simulink model "B_STUB"  (Simulink 8.1)
settings: Solver=ode1  StartTime=0.0  StopTime=1  FixedStep=Ts  MaxStep=1e-3  RelTol=1e-3
model workspace (MAT data in the model file):
  op_snapshot1 : opcond.OperatingPoint (value not decoded)
PostLoadFcn:
  | BANSHEE_init;
InitFcn:
  | BANSHEE_init;
values from neighbouring files (symbols this model uses):
  F2 = xlsread('F2_relay_banshee.xlsx')    [relay_settings_init.m]
  Ts = 100E-6    (= 0.0001)    [BANSHEE_init.m]
undefined symbols (not defined in the file or in its folder): cable_spec, Left, type, V
libraries: breaker_lib x20, relay_modbus_lib x19, rtio_generic_modbus x19, rtlab x18, cables_lib x11, transformer_lib x11, Load_lib x8, powerlib x6, ssn_lib x6, powerlib_extras x4, artemis x2, PQFV_lib x2
(part 1 of 2)
settings Model: ARTEMISmethode_block_infos=$$__separator__$$B_STUB/ARTEMIS Guide$$__separator__$$  Creator=RE25624  LastModifiedBy=re25624  BufferReuse=off
settings SolverCC: ZeroCrossAlgorithm=Adaptive
settings DataIOCC: ExternalInput=getinputstruct(op_snapshot1)  InitialState=getstatestruct(op_snapshot1)  LimitDataPoints=off  MaxDataPoints=90060  SignalLoggingSaveFormat=Dataset  SaveOutput=off  SignalLogging=off  DSMLogging=off  SaveTime=off  OutputSaveName=result
settings OptimizationCC: BlockReduction=off  OptimizeBlockIOStorage=off  BufferReuse=off  ExpressionFolding=off  LocalBlockOutputs=off
settings DebuggingCC: MaxConsecutiveZCsMsg=warning  IgnoredZcDiagnostic=none  SolverPrmCheckMsg=none  MultiTaskRateTransMsg=warning  FcnCallInpInsideContextMsg=EnableAllAsWarning  FrameProcessingCompatibilityMsg=error  ModelReferenceExtraNoncontSigs=warning  StrictBusMsg=None
settings ModelReferenceCC: UpdateModelReferenceTargets=IfOutOfDate
settings SFSimCC: SFSimEcho=off
settings GRTTargetCC: CodeReplacementLibrary=C89/C90 (ANSI)

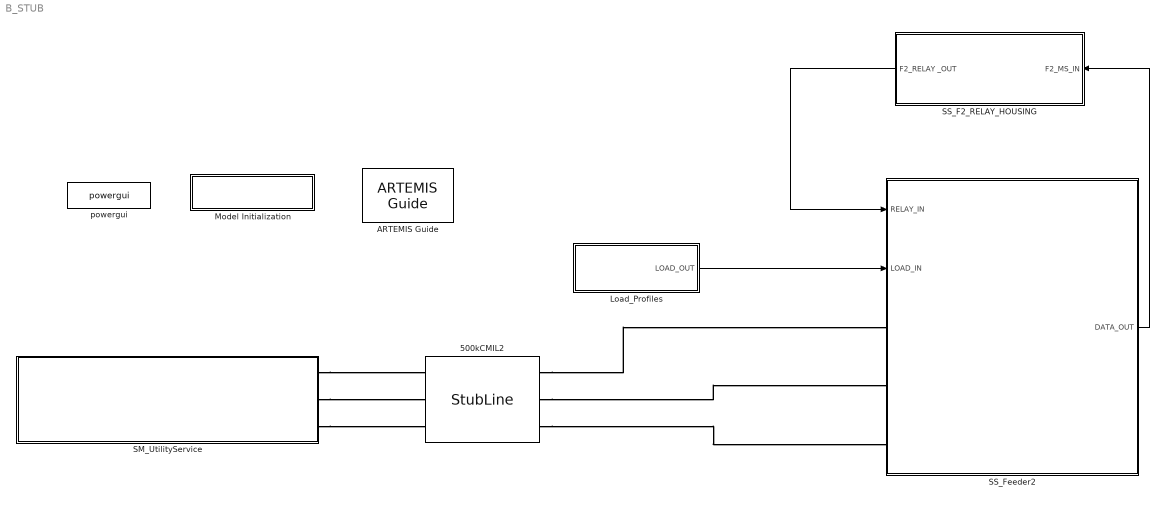
== system B_STUB ==
  500kCMIL2 : artemis/ARTEMIS/StubLine  Phases=3  pu=off  L=10000 * 9.43453e-08 / 1  Lpu=0.15  R=10000 * 2.28409e-5 / 1  Rpu=0.005  S_base=50e6/3  V_base=13.8e3/sqrt(3)  F_base=60  Ts=Ts
  ARTEMIS Guide : artemis/ARTEMIS/ARTEMIS Guide  Tag=FTSSmethode_opal_4hx0r99  Description=5.0_z1  lock=on  Ts=Ts  opt=art5  dyna=off  nb_perm=4  RT_fullcomp=off  ssn=on  ssn_itvc=off  ssn_ivic=off  ssn_ext=off  ssn_solver=Art5 with Backward Euler nodal interface  ssn_impulse=off  ssn_quasimpulse=off  ssn_impulse_loop=5  paraExtinctionThy=off  Thy_Impulse=on  dtc=Off  dtc_opt=normal  ao=on  simtype=off  ct_mac=off  lin_mov=off  lsp=[0.001 2]  spike_skip=Disabled  dtc_extra=1  dtc_sws=normal  dtc_pied=0.5  SPSRulesBlock=SPSRules  tre=on  ctmm=off  LF=off  dpl_type=ARTEMiS DPL  rlc_type=off  custom_type=off  para=on  ssn_ImpulseLoopBlockedStateUpdate=5  ssn_mov_iter_number=5  ssn_switch_iter_number=5
  Load_Profiles : Subsystem
  Model Initialization : Subsystem  AncestorBlock=artemis/Tools /Misc/Model Initialization  mask(Model Functions){InitFcnX=BANSHEE_init;, prel=off, posl=on, inif=on, strf=off}
      mask prompts: InitFcnX "Initialisation"; prel "Preload Function"; posl "PostLoad Function"; inif "InitFcn"; strf "StartFcn"
      mask init:
      | currentBlock = gcb;
      | root = bdroot(currentBlock);
      | 
      | if ~strcmp(get_param(root,'BlockDiagramType'),'library')
      |     if prel==1
      |         set_param(root, 'PreLoadFcn', InitFcnX);
      |     else
      |         set_param(root, 'PreLoadFcn', '');
      |     end
      |     if inif==1
      |         set_param(root, 'InitFcn', InitFcnX);
      |     else
      |         set_param(root, 'InitFcn', '');
      |     end
      |     if strf==1
      |         set_param(root, 'StartFcn', InitFcnX);
      |     else
      |         set_param(root, 'StartFcn', '');
      |     end
      |     if posl==1
      |         set_param(root, 'PostLoadFcn', InitFcnX);
      |     else
      |         set_param(root, 'PostLoadFcn', '');
      |     end
      | end
      | 
      | pos = get_param(currentBlock, 'Position');
      | width = pos(3) - pos(1); height = pos(4) - pos(2);
      | txt = [ upper(root) '\n' '- InitFcn. . . . . '  get_param(root, 'InitFcn') ];
      settings: CopyFcn=set_param(gcb,'LinkStatus','inactive')
      mask Display: text(5, height*0.5, txt, 'horizontalAlignment', 'left', 'verticalAlignment', 'middle') ;
  SM_UtilityService : Subsystem
  SS_F2_RELAY_HOUSING : Subsystem
  SS_Feeder2 : Subsystem
  powergui : powerlib/powergui  Priority=2  SimulationMode=Discrete  SolverType=Tustin  SampleTime=Ts  frequency=60  SPID=off  DisableSnubberDevices=off  DisableRonSwitches=off  DisableVfSwitches=off  SwTol=0  Interpol=off  DisplayEquations=off  frequencyindice=0  Pbase=100e6  ErrMax=1e-4  Iterations=50  UnitsV=kV  UnitsW=MW  FunctionMessages=off  echomessages=off  HookPort=off  EnableUseOfTLC=off  x0status=blocks  RestoreLinks=warning  ResistiveCurrentMeasurement=off  Frange=logspace(0,3,50)  Ylog=off  Xlog=off  ShowGrid=off  save=off  variable=ZData  structure=0  ZoomFFT=on  StartTime=0.0  cycles=2  DisplayStyle=off  fundamental=60  FreqAxis=off  MaxFrequency=1000  frequencyindicesteady=1  RmsSteady=1  display=off  Ts=0  methode=off
  wires:
  SS_F2_RELAY_HOUSING/1(F2_RELAY _OUT) -> SS_Feeder2/1(RELAY_IN)
  Load_Profiles/1(LOAD_OUT) -> SS_Feeder2/2(LOAD_IN)
  SS_Feeder2/1(DATA_OUT) -> SS_F2_RELAY_HOUSING/1(F2_MS_IN)
  connections:
  SM_UtilityService/RConn1 -- 500kCMIL2/LConn1
  SM_UtilityService/RConn2 -- 500kCMIL2/LConn2
  SM_UtilityService/RConn3 -- 500kCMIL2/LConn3
  500kCMIL2/RConn1 -- SS_Feeder2/LConn1
  500kCMIL2/RConn2 -- SS_Feeder2/LConn2
  500kCMIL2/RConn3 -- SS_Feeder2/LConn3

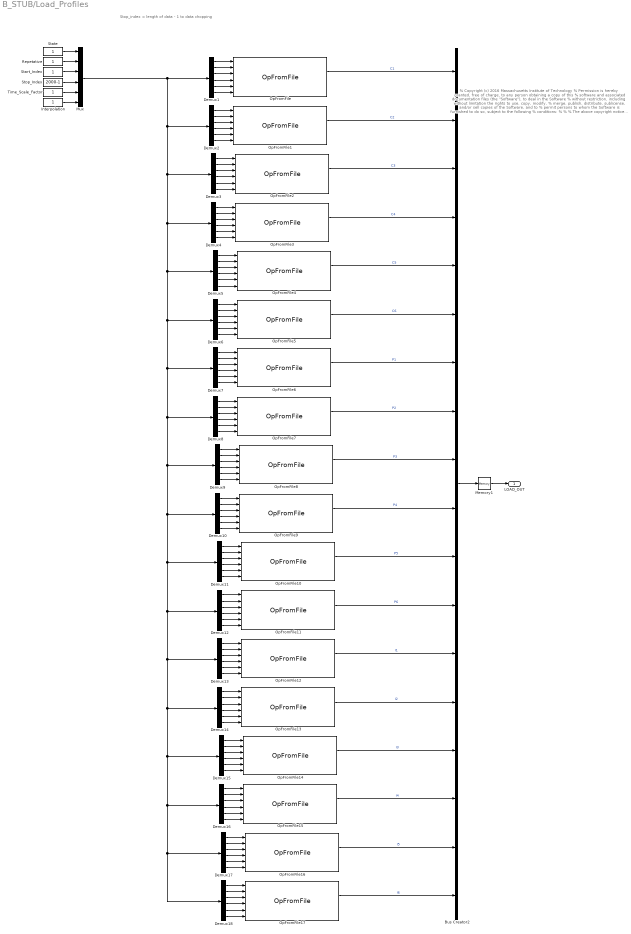
== system B_STUB/Load_Profiles ==
  note: Stop_index = length of data - 1 to data chopping
  note: % Copyright (c) 2016 Massachusetts Institute of Technology
      | % Permission is hereby granted, free of charge, to any person obtaining a copy of this
      | % software and associated documentation files (the "Software"), to deal in the Software
      | % without restriction, including without limitation the rights to use, copy, modify,
      | % merge, publish, distribute, sublicense, and/or sell copies of the Software, and to
      | % permit persons to whom the Software is furnished to do so, subject to the following
      | % conditions:
      | %
      | %
      | % The above copyright notice and this permission notice shall be included in
      | % all copies or substantial portions of the Software.
      | %
      | % THE SOFTWARE IS PROVIDED "AS IS", WITHOUT WARRANTY OF ANY KIND, EXPRESS OR IMPLIED,
      | % INCLUDING BUT NOT LIMITED TO THE WARRANTIES OF MERCHANTABILITY, FITNESS FOR A
      | % PARTICULAR PURPOSE AND NONINFRINGEMENT. IN NO EVENT SHALL THE AUTHORS OR COPYRIGHT
      | % HOLDERS BE LIABLE FOR ANY CLAIM, DAMAGES OR OTHER LIABILITY, WHETHER IN AN ACTION
      | % OF CONTRACT, TORT OR OTHERWISE, ARISING FROM, OUT OF OR IN CONNECTION WITH THE
      | % SOFTWARE OR THE USE OR OTHER DEALINGS IN THE SOFTWARE.
      | %
      | %
      | %%
  Bus Creator2 : BusCreator  Inputs=18
  Demux{1..18} (18 alike) : Demux  Outputs=6
  "Interpolation " : Constant
  Memory1 : Memory
  Mux : Mux  Inputs=6
  OpFromFile : rtlab/DataLogging/OpFromFile  filename_mode=Static (same filename all the time)  reload_mode=Next time model is paused (Real-Time)  init_file_id=0  filename=C1.mat  rtpath='./'  nrtpath='.\'  sample_time=0
  OpFromFile1 : rtlab/DataLogging/OpFromFile  filename_mode=Static (same filename all the time)  reload_mode=Next time model is paused (Real-Time)  init_file_id=0  filename=C2.mat  rtpath='./'  nrtpath='.\'  sample_time=0
  OpFromFile10 : rtlab/DataLogging/OpFromFile  filename_mode=Static (same filename all the time)  reload_mode=Next time model is paused (Real-Time)  init_file_id=0  filename=P5.mat  rtpath='./'  nrtpath='.\'  sample_time=0
  OpFromFile11 : rtlab/DataLogging/OpFromFile  filename_mode=Static (same filename all the time)  reload_mode=Next time model is paused (Real-Time)  init_file_id=0  filename=P6.mat  rtpath='./'  nrtpath='.\'  sample_time=0
  OpFromFile12 : rtlab/DataLogging/OpFromFile  filename_mode=Static (same filename all the time)  reload_mode=Next time model is paused (Real-Time)  init_file_id=0  filename=I1.mat  rtpath='./'  nrtpath='.\'  sample_time=0
  OpFromFile13 : rtlab/DataLogging/OpFromFile  filename_mode=Static (same filename all the time)  reload_mode=Next time model is paused (Real-Time)  init_file_id=0  filename=I2.mat  rtpath='./'  nrtpath='.\'  sample_time=0
  OpFromFile14 : rtlab/DataLogging/OpFromFile  filename_mode=Static (same filename all the time)  reload_mode=Next time model is paused (Real-Time)  init_file_id=0  filename=I3.mat  rtpath='./'  nrtpath='.\'  sample_time=0
  OpFromFile15 : rtlab/DataLogging/OpFromFile  filename_mode=Static (same filename all the time)  reload_mode=Next time model is paused (Real-Time)  init_file_id=0  filename=I4.mat  rtpath='./'  nrtpath='.\'  sample_time=0
  OpFromFile16 : rtlab/DataLogging/OpFromFile  filename_mode=Static (same filename all the time)  reload_mode=Next time model is paused (Real-Time)  init_file_id=0  filename=I5.mat  rtpath='./'  nrtpath='.\'  sample_time=0
  OpFromFile17 : rtlab/DataLogging/OpFromFile  filename_mode=Static (same filename all the time)  reload_mode=Next time model is paused (Real-Time)  init_file_id=0  filename=I6.mat  rtpath='./'  nrtpath='.\'  sample_time=0
  OpFromFile2 : rtlab/DataLogging/OpFromFile  filename_mode=Static (same filename all the time)  reload_mode=Next time model is paused (Real-Time)  init_file_id=0  filename=C3.mat  rtpath='./'  nrtpath='.\'  sample_time=0
  OpFromFile3 : rtlab/DataLogging/OpFromFile  filename_mode=Static (same filename all the time)  reload_mode=Next time model is paused (Real-Time)  init_file_id=0  filename=C4.mat  rtpath='./'  nrtpath='.\'  sample_time=0
  OpFromFile4 : rtlab/DataLogging/OpFromFile  filename_mode=Static (same filename all the time)  reload_mode=Next time model is paused (Real-Time)  init_file_id=0  filename=C5.mat  rtpath='./'  nrtpath='.\'  sample_time=0
  OpFromFile5 : rtlab/DataLogging/OpFromFile  filename_mode=Static (same filename all the time)  reload_mode=Next time model is paused (Real-Time)  init_file_id=0  filename=C6.mat  rtpath='./'  nrtpath='.\'  sample_time=0
  OpFromFile6 : rtlab/DataLogging/OpFromFile  filename_mode=Static (same filename all the time)  reload_mode=Next time model is paused (Real-Time)  init_file_id=0  filename=P1.mat  rtpath='./'  nrtpath='.\'  sample_time=0
  OpFromFile7 : rtlab/DataLogging/OpFromFile  filename_mode=Static (same filename all the time)  reload_mode=Next time model is paused (Real-Time)  init_file_id=0  filename=P2.mat  rtpath='./'  nrtpath='.\'  sample_time=0
  OpFromFile8 : rtlab/DataLogging/OpFromFile  filename_mode=Static (same filename all the time)  reload_mode=Next time model is paused (Real-Time)  init_file_id=0  filename=P3.mat  rtpath='./'  nrtpath='.\'  sample_time=0
  OpFromFile9 : rtlab/DataLogging/OpFromFile  filename_mode=Static (same filename all the time)  reload_mode=Next time model is paused (Real-Time)  init_file_id=0  filename=P4.mat  rtpath='./'  nrtpath='.\'  sample_time=0
  "Repetative " : Constant
  "Start_Index " : Constant
  "State " : Constant
  "Stop_Index " : Constant  Value=2000-1
  "Time_Scale_Factor " : Constant
  LOAD_OUT : Outport
  wires:
  Demux10/3 -> OpFromFile9/3
  Demux10/1 -> OpFromFile9/1
  Demux9/2 -> OpFromFile8/2
  Demux11/1 -> OpFromFile10/1
  Demux9/3 -> OpFromFile8/3
  Demux14/4 -> OpFromFile13/4
  Demux5/4 -> OpFromFile4/4
  Demux9/6 -> OpFromFile8/6
  Demux5/5 -> OpFromFile4/5
  Demux5/3 -> OpFromFile4/3
  Demux11/2 -> OpFromFile10/2
  Demux11/3 -> OpFromFile10/3
  Demux9/1 -> OpFromFile8/1
  Demux14/6 -> OpFromFile13/6
  Demux15/1 -> OpFromFile14/1
  Demux8/6 -> OpFromFile7/6
  Demux10/6 -> OpFromFile9/6
  Demux8/5 -> OpFromFile7/5
  OpFromFile3/2 -> Bus Creator2/4  "C4"
  Demux14/5 -> OpFromFile13/5
  OpFromFile5/2 -> Bus Creator2/6  "C6"
  OpFromFile4/2 -> Bus Creator2/5  "C5"
  "Interpolation "/1 -> Mux/6
  "Stop_Index "/1 -> Mux/4
  "Time_Scale_Factor "/1 -> Mux/5
  OpFromFile2/2 -> Bus Creator2/3  "C3"
  OpFromFile1/2 -> Bus Creator2/2  "C2"
  "Start_Index "/1 -> Mux/3
  OpFromFile/2 -> Bus Creator2/1  "C1"
  "State "/1 -> Mux/1
  "Repetative "/1 -> Mux/2
  Demux3/6 -> OpFromFile2/6
  Demux4/2 -> OpFromFile3/2
  Demux4/1 -> OpFromFile3/1
  Demux9/4 -> OpFromFile8/4
  Demux3/4 -> OpFromFile2/4
  Demux3/3 -> OpFromFile2/3
  Demux3/2 -> OpFromFile2/2
  Demux10/2 -> OpFromFile9/2
  Demux3/5 -> OpFromFile2/5
  Demux1/6 -> OpFromFile/6
  Demux1/5 -> OpFromFile/5
  Demux2/1 -> OpFromFile1/1
  Demux2/2 -> OpFromFile1/2
  Demux10/5 -> OpFromFile9/5
  Demux2/5 -> OpFromFile1/5
  Demux1/4 -> OpFromFile/4
  Demux2/3 -> OpFromFile1/3
  Demux2/4 -> OpFromFile1/4
  Demux3/1 -> OpFromFile2/1
  Demux10/4 -> OpFromFile9/4
  Demux2/6 -> OpFromFile1/6
  Demux1/3 -> OpFromFile/3
  Demux9/5 -> OpFromFile8/5
  Demux4/3 -> OpFromFile3/3
  Demux5/2 -> OpFromFile4/2
  Demux4/5 -> OpFromFile3/5
  Demux4/4 -> OpFromFile3/4
  Demux5/6 -> OpFromFile4/6
  Demux6/1 -> OpFromFile5/1
  Demux6/2 -> OpFromFile5/2
  Demux6/3 -> OpFromFile5/3
  Demux6/4 -> OpFromFile5/4
  Demux8/2 -> OpFromFile7/2
  Demux8/3 -> OpFromFile7/3
  Demux8/4 -> OpFromFile7/4
  Demux7/2 -> OpFromFile6/2
  Demux7/3 -> OpFromFile6/3
  Demux7/4 -> OpFromFile6/4
  Demux6/5 -> OpFromFile5/5
  Demux6/6 -> OpFromFile5/6
  Demux7/1 -> OpFromFile6/1
  Demux8/1 -> OpFromFile7/1
  Demux7/6 -> OpFromFile6/6
  Demux7/5 -> OpFromFile6/5
  Demux1/2 -> OpFromFile/2
  Demux1/1 -> OpFromFile/1
  Demux5/1 -> OpFromFile4/1
  Bus Creator2/1 -> Memory1/1
  Demux4/6 -> OpFromFile3/6
  Demux11/4 -> OpFromFile10/4
  Demux11/6 -> OpFromFile10/6
  Demux12/1 -> OpFromFile11/1
  Demux13/6 -> OpFromFile12/6
  Demux14/3 -> OpFromFile13/3
  Demux14/1 -> OpFromFile13/1
  Demux12/6 -> OpFromFile11/6
  Demux13/1 -> OpFromFile12/1
  Demux13/3 -> OpFromFile12/3
  Demux13/4 -> OpFromFile12/4
  Demux12/3 -> OpFromFile11/3
  Demux12/4 -> OpFromFile11/4
  Demux14/2 -> OpFromFile13/2
  OpFromFile11/2 -> Bus Creator2/12  "P6"
  Demux16/5 -> OpFromFile15/5
  Demux11/5 -> OpFromFile10/5
  Demux12/5 -> OpFromFile11/5
  Demux12/2 -> OpFromFile11/2
  Demux16/2 -> OpFromFile15/2
  Demux16/3 -> OpFromFile15/3
  Demux16/4 -> OpFromFile15/4
  Demux16/1 -> OpFromFile15/1
  Demux13/5 -> OpFromFile12/5
  Mux/1 -> Demux1/1, Demux2/1, Demux3/1, Demux4/1, Demux7/1, Demux8/1, Demux9/1, Demux10/1, Demux11/1, Demux12/1, Demux13/1, Demux14/1, Demux15/1, Demux16/1, Demux17/1, Demux18/1, Demux6/1, Demux5/1
  Demux15/3 -> OpFromFile14/3
  Demux15/4 -> OpFromFile14/4
  OpFromFile8/2 -> Bus Creator2/9  "P3"
  OpFromFile16/2 -> Bus Creator2/17  "I5"
  OpFromFile7/2 -> Bus Creator2/8  "P2"
  OpFromFile6/2 -> Bus Creator2/7  "P1"
  Demux18/6 -> OpFromFile17/6
  Demux18/5 -> OpFromFile17/5
  Demux18/4 -> OpFromFile17/4
  OpFromFile9/2 -> Bus Creator2/10  "P4"
  OpFromFile10/2 -> Bus Creator2/11  "P5"
  Demux15/5 -> OpFromFile14/5
  Demux15/6 -> OpFromFile14/6
  Demux18/3 -> OpFromFile17/3
  Demux17/5 -> OpFromFile16/5
  Demux18/1 -> OpFromFile17/1
  Demux18/2 -> OpFromFile17/2
  Demux17/6 -> OpFromFile16/6
  Demux17/2 -> OpFromFile16/2
  Demux17/3 -> OpFromFile16/3
  Demux17/1 -> OpFromFile16/1
  Demux17/4 -> OpFromFile16/4
  OpFromFile12/2 -> Bus Creator2/13  "I1"
  Demux15/2 -> OpFromFile14/2
  Demux13/2 -> OpFromFile12/2
  OpFromFile17/2 -> Bus Creator2/18  "I6"
  Demux16/6 -> OpFromFile15/6
  OpFromFile13/2 -> Bus Creator2/14  "I2"
  OpFromFile15/2 -> Bus Creator2/16  "I4"
  OpFromFile14/2 -> Bus Creator2/15  "I3"
  Memory1/1 -> LOAD_OUT/1

== system B_STUB/Model Initialization ==

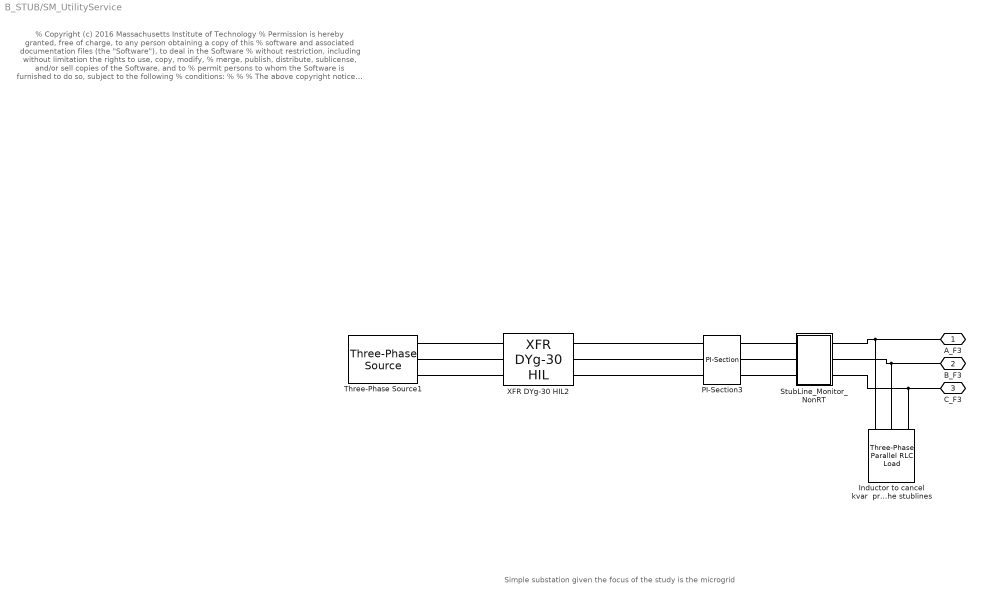
== system B_STUB/SM_UtilityService ==
  note: Simple substation given the focus of the study is the microgrid
  note: % Copyright (c) 2016 Massachusetts Institute of Technology
      | % Permission is hereby granted, free of charge, to any person obtaining a copy of this
      | % software and associated documentation files (the "Software"), to deal in the Software
      | % without restriction, including without limitation the rights to use, copy, modify,
      | % merge, publish, distribute, sublicense, and/or sell copies of the Software, and to
      | % permit persons to whom the Software is furnished to do so, subject to the following
      | % conditions:
      | %
      | %
      | % The above copyright notice and this permission notice shall be included in
      | % all copies or substantial portions of the Software.
      | %
      | % THE SOFTWARE IS PROVIDED "AS IS", WITHOUT WARRANTY OF ANY KIND, EXPRESS OR IMPLIED,
      | % INCLUDING BUT NOT LIMITED TO THE WARRANTIES OF MERCHANTABILITY, FITNESS FOR A
      | % PARTICULAR PURPOSE AND NONINFRINGEMENT. IN NO EVENT SHALL THE AUTHORS OR COPYRIGHT
      | % HOLDERS BE LIABLE FOR ANY CLAIM, DAMAGES OR OTHER LIABILITY, WHETHER IN AN ACTION
      | % OF CONTRACT, TORT OR OTHERWISE, ARISING FROM, OUT OF OR IN CONNECTION WITH THE
      | % SOFTWARE OR THE USE OR OTHER DEALINGS IN THE SOFTWARE.
      | %
      | %
      | %%
  Inductor to cancel kvar  produced by the stublines : powerlib/Elements/Three-Phase Parallel RLC Load  LConnTagsString=A|B|C  Configuration=Y (grounded)  NominalVoltage=13800  NominalFrequency=60  ActivePower=0  InductivePower=380e3  CapacitivePower=0  Measurements=None  LoadType=constant Z
  PI-Section3 : cables_lib/PI-Section  cable_spec=[cable_spec(13, :)]  line_length=500  parallel_sets=1
  StubLine_Monitor_NonRT : Subsystem  AncestorBlock=PQFV_lib/StubLine_Monitor_NonRT
  Three-Phase Source1 : powerlib/Electrical Sources/Three-Phase Source  Voltage=115000  PhaseAngle=0  Frequency=60  InternalConnection=Yg  SpecifyImpedance=on  Resistance=0.8929  Inductance=16.58e-3  ShortCircuitLevel=100e6  BaseVoltage=115000  XRratio=30  BusType=swing  Pref=0  Qref=0  Qmin=-inf  Qmax=inf
  XFR DYg-30 HIL2 : transformer_lib/XFR DYg-30 HIL  Rating=50000  Vp=115000  Vs=13800  Z=15  XR=30
  A_F3 : PMIOPort  Port=1  Side=Right
  B_F3 : PMIOPort  Port=2  Side=Right
  C_F3 : PMIOPort  Port=3  Side=Right
  connections:
  Three-Phase Source1/RConn3 -- XFR DYg-30 HIL2/LConn3
  Three-Phase Source1/RConn2 -- XFR DYg-30 HIL2/LConn2
  Three-Phase Source1/RConn1 -- XFR DYg-30 HIL2/LConn1
  StubLine_Monitor_NonRT/LConn1 -- PI-Section3/RConn1
  StubLine_Monitor_NonRT/LConn2 -- PI-Section3/RConn2
  StubLine_Monitor_NonRT/LConn3 -- PI-Section3/RConn3
  StubLine_Monitor_NonRT/RConn2 -- B_F3/RConn1 -- Inductor to cancel kvar  produced by the stublines/LConn2
  StubLine_Monitor_NonRT/RConn1 -- A_F3/RConn1 -- Inductor to cancel kvar  produced by the stublines/LConn1
  StubLine_Monitor_NonRT/RConn3 -- C_F3/RConn1 -- Inductor to cancel kvar  produced by the stublines/LConn3
  XFR DYg-30 HIL2/RConn3 -- PI-Section3/LConn3
  XFR DYg-30 HIL2/RConn2 -- PI-Section3/LConn2
  XFR DYg-30 HIL2/RConn1 -- PI-Section3/LConn1

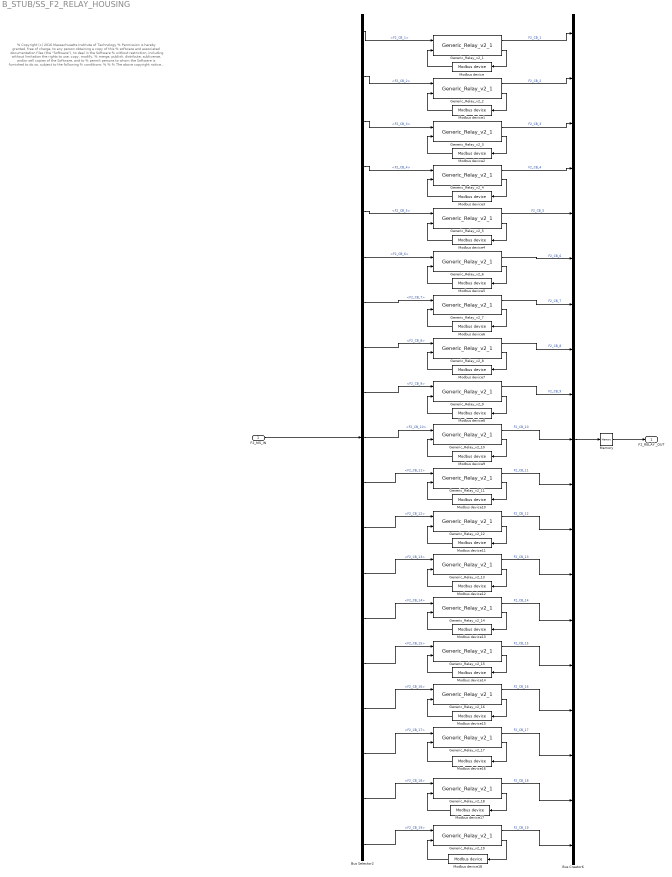
== system B_STUB/SS_F2_RELAY_HOUSING ==
  note: % Copyright (c) 2016 Massachusetts Institute of Technology
      | % Permission is hereby granted, free of charge, to any person obtaining a copy of this
      | % software and associated documentation files (the "Software"), to deal in the Software
      | % without restriction, including without limitation the rights to use, copy, modify,
      | % merge, publish, distribute, sublicense, and/or sell copies of the Software, and to
      | % permit persons to whom the Software is furnished to do so, subject to the following
      | % conditions:
      | %
      | %
      | % The above copyright notice and this permission notice shall be included in
      | % all copies or substantial portions of the Software.
      | %
      | % THE SOFTWARE IS PROVIDED "AS IS", WITHOUT WARRANTY OF ANY KIND, EXPRESS OR IMPLIED,
      | % INCLUDING BUT NOT LIMITED TO THE WARRANTIES OF MERCHANTABILITY, FITNESS FOR A
      | % PARTICULAR PURPOSE AND NONINFRINGEMENT. IN NO EVENT SHALL THE AUTHORS OR COPYRIGHT
      | % HOLDERS BE LIABLE FOR ANY CLAIM, DAMAGES OR OTHER LIABILITY, WHETHER IN AN ACTION
      | % OF CONTRACT, TORT OR OTHERWISE, ARISING FROM, OUT OF OR IN CONNECTION WITH THE
      | % SOFTWARE OR THE USE OR OTHER DEALINGS IN THE SOFTWARE.
      | %
      | %
      | %%
  F2_MS_IN : Inport
  Bus Creator6 : BusCreator  Inputs=19
  Bus Selector2 : BusSelector  OutputSignals=CB_DATA.F2_CB_1,CB_DATA.F2_CB_2,CB_DATA.F2_CB_3,CB_DATA.F2_CB_4,CB_DATA.F2_CB_5,CB_DATA.F2_CB_6,CB_DATA.F2_CB_7,CB_DATA.F2_CB_8,CB_DATA.F2_CB_9,CB_DATA.F2_CB_10,CB_DATA.F2_CB_11,CB_DATA.F2_CB_12,CB_DATA.F2_CB_13,CB_DATA.F2_CB_14,CB_DATA.F2_CB_15,CB_DATA.F2_CB_16,CB_DATA.F2_CB_17,CB_DATA.F2_CB_18,CB_DATA.F2_CB_19
  Generic_Relay_v2_1 : relay_modbus_lib/Generic_Relay_v2_1  Ts=Ts  relay_settings=[F2(1,:)]
  Generic_Relay_v2_10 : relay_modbus_lib/Generic_Relay_v2_1  Ts=Ts  relay_settings=[F2(10,:)]
  Generic_Relay_v2_11 : relay_modbus_lib/Generic_Relay_v2_1  Ts=Ts  relay_settings=[F2(11,:)]
  Generic_Relay_v2_12 : relay_modbus_lib/Generic_Relay_v2_1  Ts=Ts  relay_settings=[F2(12,:)]
  Generic_Relay_v2_13 : relay_modbus_lib/Generic_Relay_v2_1  Ts=Ts  relay_settings=[F2(13,:)]
  Generic_Relay_v2_14 : relay_modbus_lib/Generic_Relay_v2_1  Ts=Ts  relay_settings=[F2(14,:)]
  Generic_Relay_v2_15 : relay_modbus_lib/Generic_Relay_v2_1  Ts=Ts  relay_settings=[F2(15,:)]
  Generic_Relay_v2_16 : relay_modbus_lib/Generic_Relay_v2_1  Ts=Ts  relay_settings=[F2(16,:)]
  Generic_Relay_v2_17 : relay_modbus_lib/Generic_Relay_v2_1  Ts=Ts  relay_settings=[F2(17,:)]
  Generic_Relay_v2_18 : relay_modbus_lib/Generic_Relay_v2_1  Ts=Ts  relay_settings=[F2(18,:)]
  Generic_Relay_v2_19 : relay_modbus_lib/Generic_Relay_v2_1  Ts=Ts  relay_settings=[F2(19,:)]
  Generic_Relay_v2_2 : relay_modbus_lib/Generic_Relay_v2_1  Ts=Ts  relay_settings=[F2(2,:)]
  Generic_Relay_v2_3 : relay_modbus_lib/Generic_Relay_v2_1  Ts=Ts  relay_settings=[F2(3,:)]
  Generic_Relay_v2_4 : relay_modbus_lib/Generic_Relay_v2_1  Ts=Ts  relay_settings=[F2(4,:)]
  Generic_Relay_v2_5 : relay_modbus_lib/Generic_Relay_v2_1  Ts=Ts  relay_settings=[F2(5,:)]
  Generic_Relay_v2_6 : relay_modbus_lib/Generic_Relay_v2_1  Ts=Ts  relay_settings=[F2(6,:)]
  Generic_Relay_v2_7 : relay_modbus_lib/Generic_Relay_v2_1  Ts=Ts  relay_settings=[F2(7,:)]
  Generic_Relay_v2_8 : relay_modbus_lib/Generic_Relay_v2_1  Ts=Ts  relay_settings=[F2(8,:)]
  Generic_Relay_v2_9 : relay_modbus_lib/Generic_Relay_v2_1  Ts=Ts  relay_settings=[F2(9,:)]
  Memory : Memory
  Modbus device : rtio_generic_modbus/Modbus device  conf_name=F2_relay_cfg1.opal  conf_name_mask=F2_relay_cfg1.xls  sample_time=Ts
  Modbus device1 : rtio_generic_modbus/Modbus device  conf_name=F2_relay_cfg2.opal  conf_name_mask=F2_relay_cfg2.xls  sample_time=Ts
  Modbus device10 : rtio_generic_modbus/Modbus device  conf_name=F2_relay_cfg11.opal  conf_name_mask=F2_relay_cfg11.xls  sample_time=Ts
  Modbus device11 : rtio_generic_modbus/Modbus device  conf_name=F2_relay_cfg12.opal  conf_name_mask=F2_relay_cfg12.xls  sample_time=Ts
  Modbus device12 : rtio_generic_modbus/Modbus device  conf_name=F2_relay_cfg13.opal  conf_name_mask=F2_relay_cfg13.xls  sample_time=Ts
  Modbus device13 : rtio_generic_modbus/Modbus device  conf_name=F2_relay_cfg14.opal  conf_name_mask=F2_relay_cfg14.xls  sample_time=Ts
  Modbus device14 : rtio_generic_modbus/Modbus device  conf_name=F2_relay_cfg15.opal  conf_name_mask=F2_relay_cfg15.xls  sample_time=Ts
  Modbus device15 : rtio_generic_modbus/Modbus device  conf_name=F2_relay_cfg16.opal  conf_name_mask=F2_relay_cfg16.xls  sample_time=Ts
  Modbus device16 : rtio_generic_modbus/Modbus device  conf_name=F2_relay_cfg17.opal  conf_name_mask=F2_relay_cfg17.xls  sample_time=Ts
  Modbus device17 : rtio_generic_modbus/Modbus device  conf_name=F2_relay_cfg18.opal  conf_name_mask=F2_relay_cfg18.xls  sample_time=Ts
  Modbus device18 : rtio_generic_modbus/Modbus device  conf_name=F2_relay_cfg19.opal  conf_name_mask=F2_relay_cfg19.xls  sample_time=Ts
  Modbus device2 : rtio_generic_modbus/Modbus device  conf_name=F2_relay_cfg3.opal  conf_name_mask=F2_relay_cfg3.xls  sample_time=Ts
  Modbus device3 : rtio_generic_modbus/Modbus device  conf_name=F2_relay_cfg4.opal  conf_name_mask=F2_relay_cfg4.xls  sample_time=Ts
  Modbus device4 : rtio_generic_modbus/Modbus device  conf_name=F2_relay_cfg5.opal  conf_name_mask=F2_relay_cfg5.xls  sample_time=Ts
  Modbus device5 : rtio_generic_modbus/Modbus device  conf_name=F2_relay_cfg6.opal  conf_name_mask=F2_relay_cfg6.xls  sample_time=Ts
  Modbus device6 : rtio_generic_modbus/Modbus device  conf_name=F2_relay_cfg7.opal  conf_name_mask=F2_relay_cfg7.xls  sample_time=Ts
  Modbus device7 : rtio_generic_modbus/Modbus device  conf_name=F2_relay_cfg8.opal  conf_name_mask=F2_relay_cfg8.xls  sample_time=Ts
  Modbus device8 : rtio_generic_modbus/Modbus device  conf_name=F2_relay_cfg9.opal  conf_name_mask=F2_relay_cfg9.xls  sample_time=Ts
  Modbus device9 : rtio_generic_modbus/Modbus device  conf_name=F2_relay_cfg10.opal  conf_name_mask=F2_relay_cfg10.xls  sample_time=Ts
  F2_RELAY _OUT : Outport
  wires:
  Memory/1 -> F2_RELAY _OUT/1
  Bus Selector2/18 -> Generic_Relay_v2_18/1  "<F2_CB_18>"
  Bus Selector2/19 -> Generic_Relay_v2_19/1  "<F2_CB_19>"
  Generic_Relay_v2_19/1 -> Bus Creator6/19  "F2_CB_19"
  Generic_Relay_v2_18/1 -> Bus Creator6/18  "F2_CB_18"
  Generic_Relay_v2_18/2 -> Modbus device17/1
  Modbus device17/1 -> Generic_Relay_v2_18/2
  Generic_Relay_v2_19/2 -> Modbus device18/1
  Modbus device18/1 -> Generic_Relay_v2_19/2
  Bus Selector2/17 -> Generic_Relay_v2_17/1  "<F2_CB_17>"
  Generic_Relay_v2_17/1 -> Bus Creator6/17  "F2_CB_17"
  Generic_Relay_v2_6/1 -> Bus Creator6/6  "F2_CB_6"
  Generic_Relay_v2_5/1 -> Bus Creator6/5  "F2_CB_5"
  Generic_Relay_v2_4/1 -> Bus Creator6/4  "F2_CB_4"
  Generic_Relay_v2_3/1 -> Bus Creator6/3  "F2_CB_3"
  Generic_Relay_v2_2/1 -> Bus Creator6/2  "F2_CB_2"
  Generic_Relay_v2_7/1 -> Bus Creator6/7  "F2_CB_7"
  Generic_Relay_v2_8/1 -> Bus Creator6/8  "F2_CB_8"
  Generic_Relay_v2_9/1 -> Bus Creator6/9  "F2_CB_9"
  Generic_Relay_v2_10/1 -> Bus Creator6/10  "F2_CB_10"
  Generic_Relay_v2_11/1 -> Bus Creator6/11  "F2_CB_11"
  Generic_Relay_v2_16/1 -> Bus Creator6/16  "F2_CB_16"
  Generic_Relay_v2_15/1 -> Bus Creator6/15  "F2_CB_15"
  Generic_Relay_v2_14/1 -> Bus Creator6/14  "F2_CB_14"
  Generic_Relay_v2_13/1 -> Bus Creator6/13  "F2_CB_13"
  Generic_Relay_v2_12/1 -> Bus Creator6/12  "F2_CB_12"
  Bus Selector2/16 -> Generic_Relay_v2_16/1  "<F2_CB_16>"
  Bus Selector2/15 -> Generic_Relay_v2_15/1  "<F2_CB_15>"
  Bus Selector2/14 -> Generic_Relay_v2_14/1  "<F2_CB_14>"
  Bus Selector2/13 -> Generic_Relay_v2_13/1  "<F2_CB_13>"
  Bus Selector2/12 -> Generic_Relay_v2_12/1  "<F2_CB_12>"
  Bus Selector2/11 -> Generic_Relay_v2_11/1  "<F2_CB_11>"
  Bus Selector2/10 -> Generic_Relay_v2_10/1  "<F2_CB_10>"
  Bus Selector2/9 -> Generic_Relay_v2_9/1  "<F2_CB_9>"
  Bus Selector2/8 -> Generic_Relay_v2_8/1  "<F2_CB_8>"
  Bus Selector2/7 -> Generic_Relay_v2_7/1  "<F2_CB_7>"
  Bus Selector2/6 -> Generic_Relay_v2_6/1  "<F2_CB_6>"
  Bus Selector2/5 -> Generic_Relay_v2_5/1  "<F2_CB_5>"
  Bus Selector2/4 -> Generic_Relay_v2_4/1  "<F2_CB_4>"
  Bus Selector2/3 -> Generic_Relay_v2_3/1  "<F2_CB_3>"
  Bus Selector2/2 -> Generic_Relay_v2_2/1  "<F2_CB_2>"
  Generic_Relay_v2_1/1 -> Bus Creator6/1  "F2_CB_1"
  Bus Selector2/1 -> Generic_Relay_v2_1/1  "<F2_CB_1>"
  Bus Creator6/1 -> Memory/1
  Generic_Relay_v2_1/2 -> Modbus device/1
  Modbus device/1 -> Generic_Relay_v2_1/2
  Generic_Relay_v2_2/2 -> Modbus device1/1
  Modbus device1/1 -> Generic_Relay_v2_2/2
  Generic_Relay_v2_3/2 -> Modbus device2/1
  Modbus device2/1 -> Generic_Relay_v2_3/2
  Generic_Relay_v2_4/2 -> Modbus device3/1
  Modbus device3/1 -> Generic_Relay_v2_4/2
  Generic_Relay_v2_5/2 -> Modbus device4/1
  Modbus device4/1 -> Generic_Relay_v2_5/2
  Modbus device5/1 -> Generic_Relay_v2_6/2
  Generic_Relay_v2_6/2 -> Modbus device5/1
  Generic_Relay_v2_7/2 -> Modbus device6/1
  Modbus device6/1 -> Generic_Relay_v2_7/2
  Generic_Relay_v2_8/2 -> Modbus device7/1
  Modbus device7/1 -> Generic_Relay_v2_8/2
  Generic_Relay_v2_9/2 -> Modbus device8/1
  Modbus device8/1 -> Generic_Relay_v2_9/2
  Generic_Relay_v2_10/2 -> Modbus device9/1
  Modbus device9/1 -> Generic_Relay_v2_10/2
  Generic_Relay_v2_11/2 -> Modbus device10/1
  Modbus device10/1 -> Generic_Relay_v2_11/2
  Generic_Relay_v2_12/2 -> Modbus device11/1
  Modbus device11/1 -> Generic_Relay_v2_12/2
  Modbus device12/1 -> Generic_Relay_v2_13/2
  Generic_Relay_v2_13/2 -> Modbus device12/1
  Generic_Relay_v2_14/2 -> Modbus device13/1
  Modbus device13/1 -> Generic_Relay_v2_14/2
  Generic_Relay_v2_15/2 -> Modbus device14/1
  Modbus device14/1 -> Generic_Relay_v2_15/2
  Generic_Relay_v2_16/2 -> Modbus device15/1
  Modbus device15/1 -> Generic_Relay_v2_16/2
  Generic_Relay_v2_17/2 -> Modbus device16/1
  Modbus device16/1 -> Generic_Relay_v2_17/2
  F2_MS_IN/1 -> Bus Selector2/1

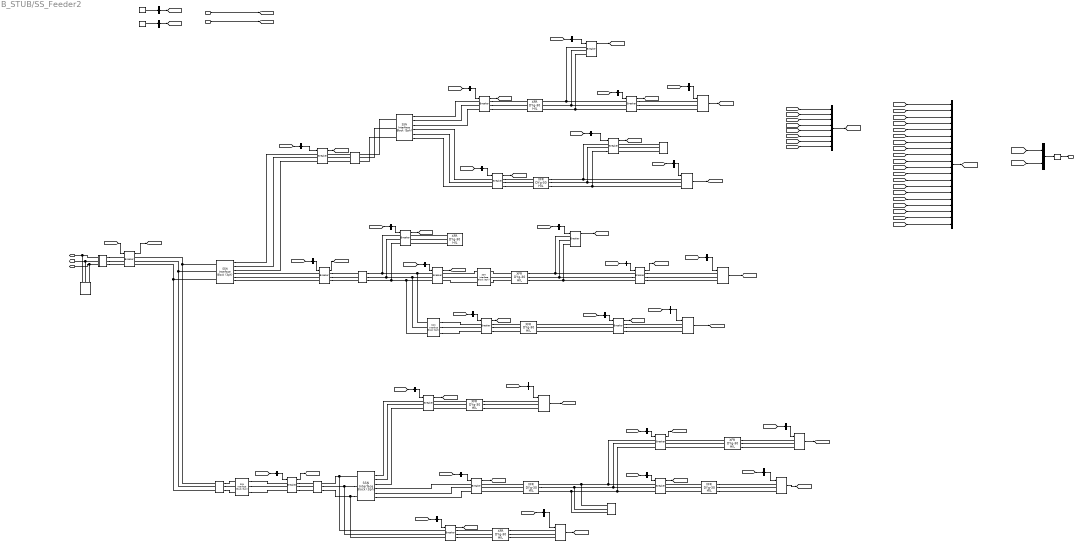
== system B_STUB/SS_Feeder2 ==
  note: Point-on-wave synchronisation voltage (3-phase) in PU - Using 13.8 kV
  note: % Copyright (c) 2016 Massachusetts Institute of Technology
      | % Permission is hereby granted, free of charge, to any person obtaining a copy of this
      | % software and associated documentation files (the "Software"), to deal in the Software
      | % without restriction, including without limitation the rights to use, copy, modify,
      | % merge, publish, distribute, sublicense, and/or sell copies of the Software, and to
      | % permit persons to whom the Software is furnished to do so, subject to the following
      | % conditions:
      | %
      | %
      | % The above copyright notice and this permission notice shall be included in
      | % all copies or substantial portions of the Software.
      | %
      | % THE SOFTWARE IS PROVIDED "AS IS", WITHOUT WARRANTY OF ANY KIND, EXPRESS OR IMPLIED,
      | % INCLUDING BUT NOT LIMITED TO THE WARRANTIES OF MERCHANTABILITY, FITNESS FOR A
      | % PARTICULAR PURPOSE AND NONINFRINGEMENT. IN NO EVENT SHALL THE AUTHORS OR COPYRIGHT
      | % HOLDERS BE LIABLE FOR ANY CLAIM, DAMAGES OR OTHER LIABILITY, WHETHER IN AN ACTION
      | % OF CONTRACT, TORT OR OTHERWISE, ARISING FROM, OUT OF OR IN CONNECTION WITH THE
      | % SOFTWARE OR THE USE OR OTHER DEALINGS IN THE SOFTWARE.
      | %
      | %
      | %%
  note: PV SYSTEM
  note: BATT SYSTEM
  note: connect to F3
  note: connect to F3
  note: connect to F3
  RELAY_IN : Inport
  LOAD_IN : Inport  Port=2
  1000 kVA1 : transformer_lib/XFR DYg-30 HIL  Rating=1000  Vp=13800  Vs=480  Z=5.56  XR=4.49
  1000 kVA2 : transformer_lib/XFR DYg-30 HIL  Rating=1000  Vp=13800  Vs=480  Z=5.56  XR=5.49
  1500 kVA : transformer_lib/XFR DYg-30 HIL  Rating=1500  Vp=13800  Vs=480  Z=5.56  XR=5.51
  2000 kVA2 : transformer_lib/XFR DYg-30 HIL  Rating=2000  Vp=13800  Vs=480  Z=5.75  XR=5.7
  2000 kVA3 : transformer_lib/XFR DYg-30 HIL  Rating=2000  Vp=13800  Vs=480  Z=5.75  XR=5.7
  2500 kVA : transformer_lib/XFR DYg-30 HIL  Rating=2500  Vp=13800  Vs=480  Z=5.56  XR=5.52
  2500 kVA1 : transformer_lib/XFR DYg-30 HIL  Rating=2500  Vp=13800  Vs=480  Z=5.56  XR=5.52
  3750 kVA : transformer_lib/XFR DYg-30 HIL  Rating=3750  Vp=13800  Vs=4160  Z=4.75  XR=11.4
  500 kVA : transformer_lib/XFR DYg-30 HIL  Rating=500  Vp=13800  Vs=208  Z=5  XR=4.9
  5000 kVA : transformer_lib/XFR DYg-30 HIL  Rating=5000  Vp=13800  Vs=480  Z=5.50  XR=5.44
  Bus Creator : BusCreator  Inputs=1
  Bus Creator1 : BusCreator  Inputs=1
  Bus Creator2 : BusCreator  Inputs=2
  Bus Creator3 : BusCreator  Inputs=8
  Bus Creator5 : BusCreator  Inputs=20
  Bus Selector1 : BusSelector  OutputSignals=F2_CB_4
  Bus Selector10 : BusSelector  OutputSignals=I4
  Bus Selector11 : BusSelector  OutputSignals=F2_CB_11
  Bus Selector12 : BusSelector  OutputSignals=F2_CB_15
  Bus Selector13 : BusSelector  OutputSignals=F2_CB_3
  Bus Selector14 : BusSelector  OutputSignals=F2_CB_14
  Bus Selector15 : BusSelector  OutputSignals=F2_CB_17
  Bus Selector16 : BusSelector  OutputSignals=F2_CB_16
  Bus Selector17 : BusSelector  OutputSignals=F2_CB_13
  Bus Selector18 : BusSelector  OutputSignals=F2_CB_10
  Bus Selector19 : BusSelector  OutputSignals=F2_CB_9
  Bus Selector2 : BusSelector  OutputSignals=F2_CB_2
  Bus Selector20 : BusSelector  OutputSignals=F2_CB_12
  Bus Selector21 : BusSelector  OutputSignals=F2_CB_5
  Bus Selector22 : BusSelector  OutputSignals=F2_CB_7
  Bus Selector23 : BusSelector  OutputSignals=F2_CB_8
  Bus Selector24 : BusSelector  OutputSignals=F2_CB_6
  Bus Selector25 : BusSelector  OutputSignals=F2_CB_1
  Bus Selector26 : BusSelector  OutputSignals=F2_CB_18
  Bus Selector27 : BusSelector  OutputSignals=F2_CB_19
  Bus Selector3 : BusSelector  OutputSignals=P5
  Bus Selector4 : BusSelector  OutputSignals=C4
  Bus Selector5 : BusSelector  OutputSignals=I5
  Bus Selector6 : BusSelector  OutputSignals=P2
  Bus Selector7 : BusSelector  OutputSignals=C3
  Bus Selector8 : BusSelector  OutputSignals=P3
  Bus Selector9 : BusSelector  OutputSignals=I3
  C1 : cables_lib/PI-Section  cable_spec=[cable_spec(11, :)]  line_length=10  parallel_sets=1
  C201 : cables_lib/PI-Section  cable_spec=[cable_spec(11, :)]  line_length=5500  parallel_sets=1
  C202 : cables_lib/PI-Section  cable_spec=[cable_spec(13, :)]  line_length=2000  parallel_sets=1
  C203 : cables_lib/PI-Section  cable_spec=[cable_spec(13, :)]  line_length=3000  parallel_sets=1
  C205 : cables_lib/PI-Section  cable_spec=[cable_spec(6, :)]  line_length=1500  parallel_sets=2
  C206 : cables_lib/PI-Section  cable_spec=[cable_spec(6, :)]  line_length=1500  parallel_sets=2
  CB closed : Constant
  CB open : Constant  Value=0
  Critical_3 : Load_lib/Dynamic_Load  V=460  Ts=Ts
  Critical_4 : Load_lib/Dynamic_Load  V=460  Ts=Ts
  F2_CB_{1..19} (19 alike) : breaker_lib/Breaker  Ts=Ts  mech_delay=cb_mech_delay
  F2_PCC : breaker_lib/Breaker  Ts=Ts  mech_delay=cb_mech_delay
  Interruptible_3 : Load_lib/Dynamic_Load  V=208  Ts=Ts
  Interruptible_4 : Load_lib/Dynamic_Load  V=460  Ts=Ts
  Interruptible_5 : Load_lib/Dynamic_Load  V=460  Ts=Ts
  Memory : Memory
  Priority_2 : Load_lib/Dynamic_Load  V=460  Ts=Ts
  Priority_3 : Load_lib/Dynamic_Load  V=460  Ts=Ts
  Priority_5 : Load_lib/Dynamic_Load  V=460  Ts=Ts
  SSN Interface Block (3ph)1 : ssn_lib/SSN Interface Block (3ph)  nb_phase=3  nb_port=3  p1_type=V-type(Left)  p2_type=V-type (Right)  p3_type=V-type (Right)  p4_type=V-type(Left)  p5_type=V-type(Left)  p6_type=V-type(Left)  p7_type=V-type(Left)  p8_type=V-type(Left)  p9_type=V-type(Left)  p10_type=V-type(Left)  p11_type=V-type(Left)  p12_type=V-type(Left)  p13_type=V-type(Left)  p14_type=V-type(Left)  p15_type=V-type(Left)  p16_type=V-type(Left)  I_port_shunt_resistance=1e9
  SSN Interface Block (3ph)10 : ssn_lib/SSN Interface Block (3ph)  nb_phase=3  nb_port=2  p1_type=V-type(Left)  p2_type=V-type (Right)  p3_type=V-type(Left)  p4_type=V-type(Left)  p5_type=V-type(Left)  p6_type=V-type(Left)  p7_type=V-type(Left)  p8_type=V-type(Left)  p9_type=V-type(Left)  p10_type=V-type(Left)  p11_type=V-type(Left)  p12_type=V-type(Left)  p13_type=V-type(Left)  p14_type=V-type(Left)  p15_type=V-type(Left)  p16_type=V-type(Left)  I_port_shunt_resistance=1e9
  SSN Interface Block (3ph)2 : ssn_lib/SSN Interface Block (3ph)  nb_phase=3  nb_port=3  p1_type=V-type(Left)  p2_type=V-type (Right)  p3_type=V-type (Right)  p4_type=V-type(Left)  p5_type=V-type(Left)  p6_type=V-type(Left)  p7_type=V-type(Left)  p8_type=V-type(Left)  p9_type=V-type(Left)  p10_type=V-type(Left)  p11_type=V-type(Left)  p12_type=V-type(Left)  p13_type=V-type(Left)  p14_type=V-type(Left)  p15_type=V-type(Left)  p16_type=V-type(Left)  I_port_shunt_resistance=1e9
  SSN Interface Block (3ph)3 : ssn_lib/SSN Interface Block (3ph)  nb_phase=3  nb_port=2  p1_type=V-type(Left)  p2_type=V-type (Right)  p3_type=V-type(Left)  p4_type=V-type(Left)  p5_type=V-type(Left)  p6_type=V-type(Left)  p7_type=V-type(Left)  p8_type=V-type(Left)  p9_type=V-type(Left)  p10_type=V-type(Left)  p11_type=V-type(Left)  p12_type=V-type(Left)  p13_type=V-type(Left)  p14_type=V-type(Left)  p15_type=V-type(Left)  p16_type=V-type(Left)  I_port_shunt_resistance=1e9
  SSN Interface Block (3ph)4 : ssn_lib/SSN Interface Block (3ph)  nb_phase=3  nb_port=3  p1_type=V-type(Left)  p2_type=V-type (Right)  p3_type=V-type (Right)  p4_type=V-type(Left)  p5_type=V-type(Left)  p6_type=V-type(Left)  p7_type=V-type(Left)  p8_type=V-type(Left)  p9_type=V-type(Left)  p10_type=V-type(Left)  p11_type=V-type(Left)  p12_type=V-type(Left)  p13_type=V-type(Left)  p14_type=V-type(Left)  p15_type=V-type(Left)  p16_type=V-type(Left)  I_port_shunt_resistance=1e9
  SSN Interface Block (3ph)9 : ssn_lib/SSN Interface Block (3ph)  nb_phase=3  nb_port=2  p1_type=V-type(Left)  p2_type=V-type (Right)  p3_type=V-type(Left)  p4_type=V-type(Left)  p5_type=V-type(Left)  p6_type=V-type(Left)  p7_type=V-type(Left)  p8_type=V-type(Left)  p9_type=V-type(Left)  p10_type=V-type(Left)  p11_type=V-type(Left)  p12_type=V-type(Left)  p13_type=V-type(Left)  p14_type=V-type(Left)  p15_type=V-type(Left)  p16_type=V-type(Left)  I_port_shunt_resistance=1e9
  StubLine_Monitor_NonRT : Subsystem  AncestorBlock=PQFV_lib/StubLine_Monitor_NonRT
  Three-Phase Parallel RLC Load : powerlib/Elements/Three-Phase Parallel RLC Load  LConnTagsString=A|B|C  Configuration=Y (grounded)  NominalVoltage=13800  NominalFrequency=60  ActivePower=0  InductivePower=380e3  CapacitivePower=0  Measurements=None  LoadType=constant Z
  A_PCC : PMIOPort  Port=1  Side=Left
  B_PCC : PMIOPort  Port=2  Side=Left
  C_PCC : PMIOPort  Port=3  Side=Left
  DATA_OUT : Outport
  wires:
  [LOAD_DATA] -> Bus Creator2/2  "LOAD_DATA"
  [CB_DATA] -> Bus Creator2/1  "CB_DATA"
  Bus Creator5/1 -> [CB_DATA]
  Bus Creator2/1 -> Memory/1
  Memory/1 -> DATA_OUT/1
  Bus Selector27/1 -> F2_CB_19/1  "<F2_CB_19>"
  [RELAY_IN] -> Bus Selector27/1
  F2_CB_19/1 -> [F2_CB_19]
  [F2_CB_19] -> Bus Creator5/19  "F2_CB_19"
  [F2_CB_18] -> Bus Creator5/18  "F2_CB_18"
  Bus Selector26/1 -> F2_CB_18/1  "<F2_CB_18>"
  [RELAY_IN] -> Bus Selector26/1
  F2_CB_18/1 -> [F2_CB_18]
  Bus Selector1/1 -> F2_CB_4/1  "<F2_CB_4>"
  [RELAY_IN] -> Bus Selector1/1
  F2_CB_4/1 -> [F2_CB_4]
  [F2_PCC] -> Bus Creator5/20  "F2_PCC"
  F2_PCC/1 -> [F2_PCC]
  F2_CB_16/1 -> [F2_CB_16]
  F2_CB_12/1 -> [F2_CB_12]
  Bus Selector15/1 -> F2_CB_17/1  "<F2_CB_17>"
  [F2_CB_17] -> Bus Creator5/17  "F2_CB_17"
  Bus Selector23/1 -> F2_CB_8/1  "<F2_CB_8>"
  Bus Selector24/1 -> F2_CB_6/1  "<F2_CB_6>"
  Bus Selector22/1 -> F2_CB_7/1  "<F2_CB_7>"
  Bus Selector21/1 -> F2_CB_5/1  "<F2_CB_5>"
  Bus Selector25/1 -> F2_CB_1/1  "<F2_CB_1>"
  Bus Selector12/1 -> F2_CB_15/1  "<F2_CB_15>"
  Bus Selector16/1 -> F2_CB_16/1  "<F2_CB_16>"
  Bus Selector14/1 -> F2_CB_14/1  "<F2_CB_14>"
  Bus Selector20/1 -> F2_CB_12/1  "<F2_CB_12>"
  Bus Selector17/1 -> F2_CB_13/1  "<F2_CB_13>"
  Bus Selector19/1 -> F2_CB_9/1  "<F2_CB_9>"
  Bus Selector18/1 -> F2_CB_10/1  "<F2_CB_10>"
  Bus Selector11/1 -> F2_CB_11/1  "<F2_CB_11>"
  Bus Selector2/1 -> F2_CB_2/1  "<F2_CB_2>"
  [RELAY_IN] -> Bus Selector25/1
  [RELAY_IN] -> Bus Selector24/1
  [RELAY_IN] -> Bus Selector23/1
  [RELAY_IN] -> Bus Selector22/1
  [RELAY_IN] -> Bus Selector21/1
  [RELAY_IN] -> Bus Selector20/1
  [RELAY_IN] -> Bus Selector19/1
  [RELAY_IN] -> Bus Selector18/1
  [RELAY_IN] -> Bus Selector17/1
  [RELAY_IN] -> Bus Selector16/1
  [RELAY_IN] -> Bus Selector15/1
  [RELAY_IN] -> Bus Selector14/1
  [RELAY_IN] -> Bus Selector12/1
  [RELAY_IN] -> Bus Selector11/1
  [RELAY_IN] -> Bus Selector2/1
  [RELAY_IN] -> Bus Selector13/1
  Bus Selector13/1 -> F2_CB_3/1  "<F2_CB_3>"
  RELAY_IN/1 -> [RELAY_IN]
  [F2_CB_16] -> Bus Creator5/16  "F2_CB_16"
  [F2_CB_15] -> Bus Creator5/15  "F2_CB_15"
  [F2_CB_13] -> Bus Creator5/13  "F2_CB_13"
  [F2_CB_10] -> Bus Creator5/10  "F2_CB_10"
  [F2_CB_12] -> Bus Creator5/12  "F2_CB_12"
  [F2_CB_8] -> Bus Creator5/8  "F2_CB_8"
  [F2_CB_5] -> Bus Creator5/5  "F2_CB_5"
  [F2_CB_14] -> Bus Creator5/14  "F2_CB_14"
  [F2_CB_11] -> Bus Creator5/11  "F2_CB_11"
  [F2_CB_7] -> Bus Creator5/7  "F2_CB_7"
  [F2_CB_9] -> Bus Creator5/9  "F2_CB_9"
  [F2_CB_4] -> Bus Creator5/4  "F2_CB_4"
  [F2_CB_6] -> Bus Creator5/6  "F2_CB_6"
  [F2_CB_3] -> Bus Creator5/3  "F2_CB_3"
  [F2_CB_2] -> Bus Creator5/2  "F2_CB_2"
  [F2_CB_1] -> Bus Creator5/1  "F2_CB_1"
  F2_CB_13/1 -> [F2_CB_13]
  F2_CB_10/1 -> [F2_CB_10]
  F2_CB_14/1 -> [F2_CB_14]
  F2_CB_17/1 -> [F2_CB_17]
  F2_CB_15/1 -> [F2_CB_15]
  F2_CB_11/1 -> [F2_CB_11]
  F2_CB_3/1 -> [F2_CB_3]
  F2_CB_9/1 -> [F2_CB_9]
  F2_CB_8/1 -> [F2_CB_8]
  F2_CB_5/1 -> [F2_CB_5]
  F2_CB_7/1 -> [F2_CB_7]
  F2_CB_6/1 -> [F2_CB_6]
  F2_CB_1/1 -> [F2_CB_1]
  F2_CB_2/1 -> [F2_CB_2]
  [LOAD_P5] -> Bus Creator3/8  "F2_P5"
  [LOAD_P3] -> Bus Creator3/7  "F2_P3"
  [LOAD_I3] -> Bus Creator3/3  "F2_I3"
  [LOAD_C4] -> Bus Creator3/2  "F2_C4"
  [LOAD_I5] -> Bus Creator3/5  "F2_I5"
  [LOAD_P2] -> Bus Creator3/6  "F2_P2"
  [LOAD_I4] -> Bus Creator3/4  "F2_I4"
  Bus Creator3/1 -> [LOAD_DATA]  "LOAD"
  [LOAD_C3] -> Bus Creator3/1  "F2_C3"
  Interruptible_4/1 -> [LOAD_I4]
  Priority_3/1 -> [LOAD_P3]
  Interruptible_3/1 -> [LOAD_I3]
  Critical_3/1 -> [LOAD_C3]
  Priority_2/1 -> [LOAD_P2]
  Interruptible_5/1 -> [LOAD_I5]
  Priority_5/1 -> [LOAD_P5]
  Critical_4/1 -> [LOAD_C4]
  Bus Selector9/1 -> Interruptible_3/1  "<I3>"
  Bus Selector10/1 -> Interruptible_4/1  "<I4>"
  Bus Selector8/1 -> Priority_3/1  "<P3>"
  Bus Selector7/1 -> Critical_3/1  "<C3>"
  Bus Selector6/1 -> Priority_2/1  "<P2>"
  Bus Selector5/1 -> Interruptible_5/1  "<I5>"
  Bus Selector4/1 -> Critical_4/1  "<C4>"
  Bus Selector3/1 -> Priority_5/1  "<P5>"
  [LOAD_IN] -> Bus Selector10/1
  [LOAD_IN] -> Bus Selector9/1
  [LOAD_IN] -> Bus Selector8/1
  [LOAD_IN] -> Bus Selector7/1
  [LOAD_IN] -> Bus Selector6/1
  [LOAD_IN] -> Bus Selector5/1
  [LOAD_IN] -> Bus Selector4/1
  [LOAD_IN] -> Bus Selector3/1
  LOAD_IN/1 -> [LOAD_IN]
  CB open/1 -> Bus Creator1/1  "Logic_trip"
  Bus Creator1/1 -> [cb_o]
  CB closed/1 -> Bus Creator/1  "Logic_trip"
  Bus Creator/1 -> [cb_c]
  [cb_c] -> F2_PCC/1
  connections:
  StubLine_Monitor_NonRT/LConn3 -- Three-Phase Parallel RLC Load/LConn3 -- C_PCC/RConn1
  StubLine_Monitor_NonRT/LConn1 -- Three-Phase Parallel RLC Load/LConn1 -- A_PCC/RConn1
  StubLine_Monitor_NonRT/LConn2 -- Three-Phase Parallel RLC Load/LConn2 -- B_PCC/RConn1
  500 kVA/RConn1 -- Interruptible_3/LConn1
  500 kVA/RConn3 -- Interruptible_3/LConn3
  500 kVA/RConn2 -- Interruptible_3/LConn2
  1000 kVA2/RConn3 -- Interruptible_4/LConn3
  1000 kVA2/RConn2 -- Interruptible_4/LConn2
  1000 kVA2/RConn1 -- Interruptible_4/LConn1
  2500 kVA/RConn2 -- Critical_3/LConn2
  2500 kVA/RConn3 -- Critical_3/LConn3
  2500 kVA/RConn1 -- Critical_3/LConn1
  C1/RConn3 -- SSN Interface Block (3ph)10/LConn3
  C1/RConn1 -- SSN Interface Block (3ph)10/LConn1
  C1/RConn2 -- SSN Interface Block (3ph)10/LConn2
  SSN Interface Block (3ph)10/RConn3 -- F2_CB_1/LConn3
  SSN Interface Block (3ph)10/RConn2 -- F2_CB_1/LConn2
  SSN Interface Block (3ph)10/RConn1 -- F2_CB_1/LConn1
  SSN Interface Block (3ph)1/RConn6 -- F2_CB_7/LConn3
  SSN Interface Block (3ph)1/RConn5 -- F2_CB_7/LConn2
  SSN Interface Block (3ph)1/RConn4 -- F2_CB_7/LConn1
  SSN Interface Block (3ph)1/LConn3 -- F2_CB_6/LConn3 -- C201/RConn3
  C201/RConn1 -- F2_CB_6/LConn1 -- SSN Interface Block (3ph)1/LConn1
  SSN Interface Block (3ph)1/LConn2 -- F2_CB_6/LConn2 -- C201/RConn2
  F2_CB_1/RConn3 -- C201/LConn3
  F2_CB_1/RConn2 -- C201/LConn2
  F2_CB_1/RConn1 -- C201/LConn1
  SSN Interface Block (3ph)1/RConn1 -- F2_CB_5/LConn1
  SSN Interface Block (3ph)1/RConn3 -- F2_CB_5/LConn3
  SSN Interface Block (3ph)2/RConn4 -- F2_CB_14/LConn1
  SSN Interface Block (3ph)2/RConn5 -- F2_CB_14/LConn2
  SSN Interface Block (3ph)2/RConn6 -- F2_CB_14/LConn3
  SSN Interface Block (3ph)2/RConn3 -- F2_CB_15/LConn3
  SSN Interface Block (3ph)2/RConn2 -- F2_CB_15/LConn2
  SSN Interface Block (3ph)2/RConn1 -- F2_CB_15/LConn1
  F2_CB_2/RConn3 -- C202/LConn3
  F2_CB_2/RConn1 -- C202/LConn1
  F2_CB_2/RConn2 -- C202/LConn2
  SSN Interface Block (3ph)4/RConn4 -- F2_CB_2/LConn1
  SSN Interface Block (3ph)4/RConn6 -- F2_CB_2/LConn3
  SSN Interface Block (3ph)4/RConn5 -- F2_CB_2/LConn2
  1500 kVA/LConn1 -- F2_CB_4/RConn1
  1500 kVA/LConn2 -- F2_CB_4/RConn2
  1500 kVA/LConn3 -- F2_CB_4/RConn3
  1500 kVA/RConn1 -- Priority_3/LConn1
  1500 kVA/RConn2 -- Priority_3/LConn2
  1500 kVA/RConn3 -- Priority_3/LConn3
  C205/LConn2 -- F2_CB_17/RConn2
  C205/LConn1 -- F2_CB_17/RConn1
  C205/LConn3 -- F2_CB_17/RConn3
  SSN Interface Block (3ph)3/RConn1 -- F2_CB_9/LConn1
  SSN Interface Block (3ph)3/RConn3 -- F2_CB_9/LConn3
  SSN Interface Block (3ph)3/RConn2 -- F2_CB_9/LConn2
  F2_CB_19/RConn3 -- Priority_2/LConn3
  F2_CB_19/RConn2 -- Priority_2/LConn2
  F2_CB_19/RConn1 -- Priority_2/LConn1
  F2_CB_18/RConn3 -- Priority_5/LConn3
  F2_CB_18/RConn2 -- Priority_5/LConn2
  F2_CB_18/RConn1 -- Priority_5/LConn1
  F2_CB_19/LConn3 -- 2500 kVA1/RConn3
  F2_CB_19/LConn1 -- 2500 kVA1/RConn1
  F2_CB_9/RConn2 -- 2500 kVA1/LConn2
  F2_PCC/RConn3 -- SSN Interface Block (3ph)4/LConn3 -- C1/LConn3
  C1/LConn2 -- F2_PCC/RConn2 -- SSN Interface Block (3ph)4/LConn2
  F2_CB_6/RConn1 -- 500 kVA/LConn1
  F2_CB_15/RConn2 -- 2000 kVA3/LConn2
  C202/RConn1 -- F2_CB_11/LConn1 -- F2_CB_10/LConn1 -- SSN Interface Block (3ph)3/LConn1
  3750 kVA/LConn1 -- F2_CB_7/RConn1
  3750 kVA/LConn2 -- F2_CB_7/RConn2
  2000 kVA2/RConn2 -- F2_CB_17/LConn2 -- Critical_4/LConn2
  5000 kVA/LConn3 -- F2_CB_11/RConn3
  C203/LConn2 -- F2_CB_3/RConn2
  F2_CB_19/LConn2 -- 2500 kVA1/RConn2
  F2_CB_9/RConn1 -- 2500 kVA1/LConn1
  F2_CB_15/RConn3 -- 2000 kVA3/LConn3
  5000 kVA/LConn1 -- F2_CB_11/RConn1
  F2_CB_17/LConn3 -- 2000 kVA2/RConn3 -- Critical_4/LConn3
  F2_CB_15/RConn1 -- 2000 kVA3/LConn1
  F2_CB_14/RConn1 -- 2000 kVA2/LConn1
  SSN Interface Block (3ph)9/LConn1 -- F2_CB_10/RConn1
  2000 kVA3/RConn1 -- F2_CB_18/LConn1 -- F2_CB_16/LConn1
  2500 kVA/LConn2 -- F2_CB_5/RConn2
  2500 kVA/LConn3 -- F2_CB_5/RConn3
  2500 kVA/LConn1 -- F2_CB_5/RConn1
  SSN Interface Block (3ph)9/LConn2 -- F2_CB_10/RConn2
  C203/LConn1 -- F2_CB_3/RConn1
  C203/LConn3 -- F2_CB_3/RConn3
  3750 kVA/LConn3 -- F2_CB_7/RConn3
  C1/LConn1 -- F2_PCC/RConn1 -- SSN Interface Block (3ph)4/LConn1
  C202/RConn2 -- F2_CB_11/LConn2 -- SSN Interface Block (3ph)3/LConn2 -- F2_CB_10/LConn2
  2000 kVA2/RConn1 -- F2_CB_17/LConn1 -- Critical_4/LConn1
  5000 kVA/LConn2 -- F2_CB_11/RConn2
  F2_CB_18/LConn3 -- 2000 kVA3/RConn3 -- F2_CB_16/LConn3
  F2_CB_6/RConn3 -- 500 kVA/LConn3
  C202/RConn3 -- F2_CB_11/LConn3 -- F2_CB_10/LConn3 -- SSN Interface Block (3ph)3/LConn3
  F2_CB_9/RConn3 -- 2500 kVA1/LConn3
  SSN Interface Block (3ph)9/LConn3 -- F2_CB_10/RConn3
  F2_CB_6/RConn2 -- 500 kVA/LConn2
  F2_CB_14/RConn2 -- 2000 kVA2/LConn2
  F2_CB_18/LConn2 -- 2000 kVA3/RConn2 -- F2_CB_16/LConn2
  F2_CB_14/RConn3 -- 2000 kVA2/LConn3
  SSN Interface Block (3ph)4/RConn2 -- F2_CB_3/LConn2
  SSN Interface Block (3ph)4/RConn1 -- F2_CB_3/LConn1
  SSN Interface Block (3ph)4/RConn3 -- F2_CB_3/LConn3
  SSN Interface Block (3ph)1/RConn2 -- F2_CB_5/LConn2
  1000 kVA2/LConn2 -- F2_CB_8/RConn2
  1000 kVA2/LConn1 -- F2_CB_8/RConn1
  1000 kVA2/LConn3 -- F2_CB_8/RConn3
  F2_CB_4/LConn1 -- F2_CB_8/LConn1 -- C206/LConn1 -- 3750 kVA/RConn1
  F2_CB_4/LConn3 -- F2_CB_8/LConn3 -- C206/LConn3 -- 3750 kVA/RConn3
  F2_CB_8/LConn2 -- C206/LConn2 -- 3750 kVA/RConn2 -- F2_CB_4/LConn2
  1000 kVA1/LConn2 -- SSN Interface Block (3ph)9/RConn2
  1000 kVA1/LConn3 -- SSN Interface Block (3ph)9/RConn3
  1000 kVA1/LConn1 -- SSN Interface Block (3ph)9/RConn1
  F2_CB_12/RConn1 -- Interruptible_5/LConn1
  F2_CB_12/RConn2 -- Interruptible_5/LConn2
  F2_CB_12/RConn3 -- Interruptible_5/LConn3
  1000 kVA1/RConn3 -- F2_CB_12/LConn3 -- F2_CB_13/LConn3
  F2_CB_12/LConn2 -- 1000 kVA1/RConn2 -- F2_CB_13/LConn2
  1000 kVA1/RConn1 -- F2_CB_12/LConn1 -- F2_CB_13/LConn1
  SSN Interface Block (3ph)2/LConn3 -- C203/RConn3
  SSN Interface Block (3ph)2/LConn2 -- C203/RConn2
  SSN Interface Block (3ph)2/LConn1 -- C203/RConn1
  StubLine_Monitor_NonRT/RConn3 -- F2_PCC/LConn3
  StubLine_Monitor_NonRT/RConn2 -- F2_PCC/LConn2
  StubLine_Monitor_NonRT/RConn1 -- F2_PCC/LConn1

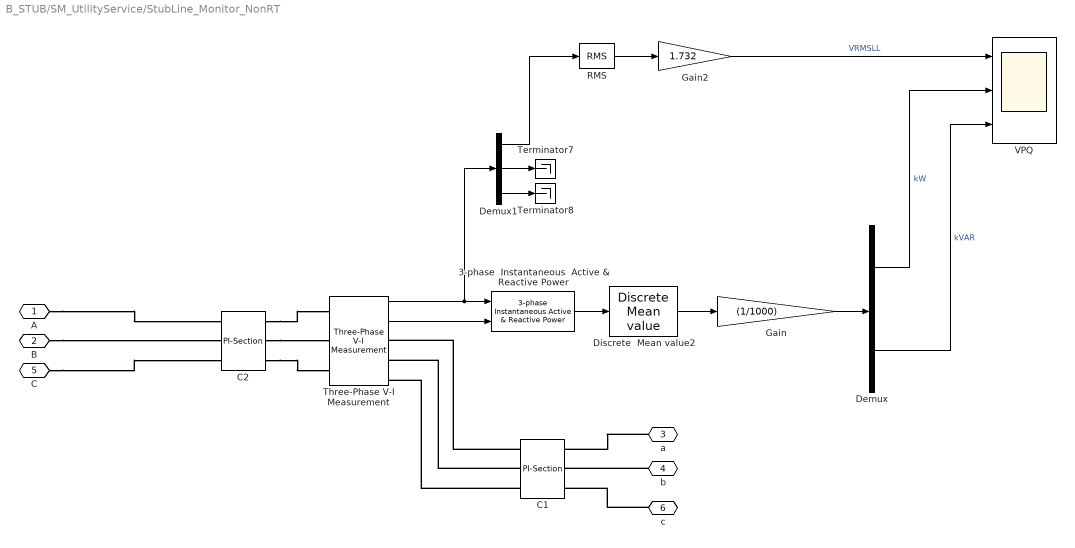
== system B_STUB/SM_UtilityService/StubLine_Monitor_NonRT ==
  3-phase  Instantaneous  Active & Reactive Power : powerlib_extras/Measurements/3-phase  Instantaneous  Active & Reactive Power
  C1 : cables_lib/PI-Section  cable_spec=[cable_spec(13, :)]  line_length=2500  parallel_sets=1
  C2 : cables_lib/PI-Section  cable_spec=[cable_spec(13, :)]  line_length=2500  parallel_sets=1
  Demux : Demux  Outputs=2
  Demux1 : Demux  Outputs=3
  Discrete  Mean value2 : powerlib_extras/Discrete Measurements/Discrete  Mean value  Freq=60  Vinit=0  Ts=Ts
  Gain : Gain  Gain=(1/1000)
  Gain2 : Gain  Gain=1.732
  RMS : PQFV_lib/PQFV/RMS
  Terminator7 : Terminator
  Terminator8 : Terminator
  Three-Phase V-I Measurement : powerlib/Measurements/Three-Phase V-I Measurement  VoltageMeasurement=phase-to-ground  SetLabelV=off  LabelV=Vabc  Vpu=off  VpuLL=off  CurrentMeasurement=yes  SetLabelI=off  LabelI=Iabc  Ipu=off  Pbase=100e6  Vbase=500e3  OutputType=Complex  PhasorSimulation=off  PSBequivalent=0
  VPQ : Scope  NumInputPorts=3
      settings: TimeRange=6  YMin=0~-500~-2300  YMax=15000~4000~0  SaveName=ScopeData2
  A : PMIOPort  Port=1  Side=Left
  B : PMIOPort  Port=2  Side=Left
  a : PMIOPort  Port=3  Side=Right
  b : PMIOPort  Port=4  Side=Right
  C : PMIOPort  Port=5  Side=Left
  c : PMIOPort  Port=6  Side=Right
  wires:
  Demux/2 -> VPQ/3  "kVAR"
  Demux/1 -> VPQ/2  "kW"
  Gain2/1 -> VPQ/1  "VRMSLL"
  Three-Phase V-I Measurement/2 -> 3-phase  Instantaneous  Active & Reactive Power/2
  Three-Phase V-I Measurement/1 -> 3-phase  Instantaneous  Active & Reactive Power/1, Demux1/1
  Discrete  Mean value2/1 -> Gain/1
  3-phase  Instantaneous  Active & Reactive Power/1 -> Discrete  Mean value2/1
  Demux1/1 -> RMS/1
  Demux1/2 -> Terminator7/1
  Demux1/3 -> Terminator8/1
  RMS/1 -> Gain2/1
  Gain/1 -> Demux/1
  connections:
  b/RConn1 -- C1/RConn2
  a/RConn1 -- C1/RConn1
  c/RConn1 -- C1/RConn3
  C1/LConn1 -- Three-Phase V-I Measurement/RConn1
  C1/LConn3 -- Three-Phase V-I Measurement/RConn3
  C1/LConn2 -- Three-Phase V-I Measurement/RConn2
  C2/RConn2 -- Three-Phase V-I Measurement/LConn2
  C2/RConn1 -- Three-Phase V-I Measurement/LConn1
  C2/RConn3 -- Three-Phase V-I Measurement/LConn3
  B/RConn1 -- C2/LConn2
  A/RConn1 -- C2/LConn1
  C/RConn1 -- C2/LConn3
